simulink model "reglertest2"  (Simulink 7.4)
settings: Solver=ode23  StartTime=0.0  StopTime=1000  MaxStep=0.01  RelTol=1e-3
values from neighbouring files (symbols this model uses):
  KD = polyCOGx    [automatic_controller_2_NOPDT.m]    (also in automatic_controller_2_NOPDT_dycops.m; automatic_controller_NOPDT.m; manual_controller_NOPDT.m = KDa; stable_regions_PID5.m = optimalpolyCOGx)
  KI = polyCOGy    [automatic_controller_2_NOPDT.m]    (also in automatic_controller_2_NOPDT_dycops.m; automatic_controller_NOPDT.m; manual_controller_NOPDT.m = KIa; stable_regions_PID5.m = optimalpolyCOGy)
  KP = KPAmax    [automatic_controller_2_NOPDT.m]    (also in automatic_controller_2_NOPDT_dycops.m; automatic_controller_NOPDT.m = 0.05*KPmax; calc_max_polytope.m = KPvec(i); calc_max_polytope_NO.m = KPvec(i))
  L1 = get(Gref1,'OutputDelay')    [automatic_controller_2_NOPDT.m]    (also in automatic_controller_2_NOPDT_dycops.m)
undefined symbols (not defined in the file or in its folder): Ds1, Ns1
libraries: simulink x3
settings Model: Creator=sle  LastModifiedBy=sle

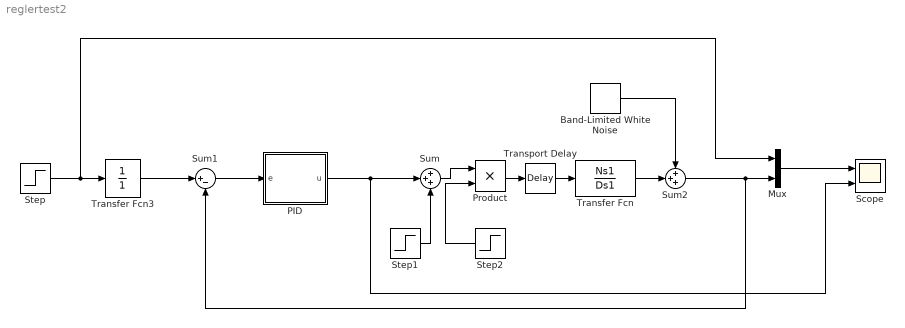
== system reglertest2 ==
  Band-Limited White Noise : simulink/Sources/Band-Limited White Noise  SystemSampleTime=-1  Cov=[0.00001]  Ts=0.1  seed=[23341]
  Mux : Mux  Inputs=2
  PID : Subsystem  mask{KP=KP, KI=KI, KD=KD, Tf=10, OG=900, UG=0}
      mask prompts: Tf "Filterzeitkonstante Tf"; OG "AntiWindup Obergrenze"; UG "AntiWindup Untergrenze"
  Product : Product  OutDataType=fixdt(1, 16)  OutScaling=2^0  RndMeth=Zero
  Scope : Scope  NumInputPorts=2
      settings: YMin=-5~-5  YMax=5~5
  Step : Step  Time=700  Before=1  After=0.5  SampleTime=0
  Step1 : Step  Time=300  After=0.1  SampleTime=0
  Step2 : Step  Time=500  Before=1  After=2  SampleTime=0
  Sum : Sum  Inputs=+++  OutDataType=fixdt(1, 16)  OutScaling=2^0
  Sum1 : Sum  Inputs=|+-  OutDataType=fixdt(1, 16)  OutScaling=2^0
  Sum2 : Sum  Inputs=+++  OutDataType=fixdt(1, 16)  OutScaling=2^0
  Transfer Fcn : TransferFcn  Numerator=Ns1  Denominator=Ds1
  Transfer Fcn3 : TransferFcn  Numerator=1  Denominator=1
  Transport Delay : TransportDelay  DelayTime=L1
  wires:
  Transport Delay/1 -> Transfer Fcn/1
  PID/1(u) -> Sum/2, Scope/2
  Step/1 -> Transfer Fcn3/1, Mux/1
  Mux/1 -> Scope/1
  Step1/1 -> Sum/3
  Sum1/1 -> PID/1(e)
  Transfer Fcn/1 -> Sum2/2
  Sum2/1 -> Mux/2, Sum1/2
  Band-Limited White Noise/1 -> Sum2/1
  Transfer Fcn3/1 -> Sum1/1
  Product/1 -> Transport Delay/1
  Sum/1 -> Product/1
  Step2/1 -> Product/2

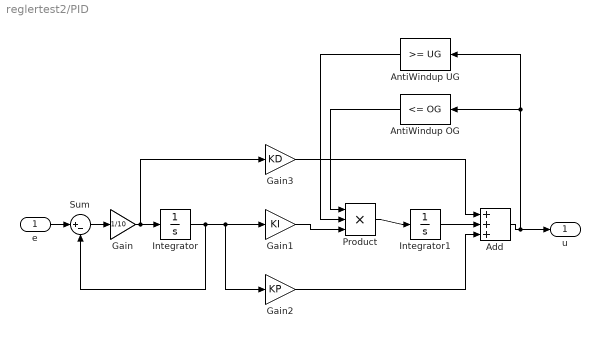
== system reglertest2/PID ==
  e : Inport  OutDataType=fixdt(1, 16)  OutScaling=2^0
  Add : Sum  Inputs=+++  OutDataType=fixdt(1, 16)  OutScaling=2^-10
  AntiWindup OG : simulink/Logic and Bit Operations/Compare To Constant  SystemSampleTime=-1  relop=<=  const=OG  LogicOutDataTypeMode=uint8  ZeroCross=off
  AntiWindup UG : simulink/Logic and Bit Operations/Compare To Constant  SystemSampleTime=-1  relop=>=  const=UG  LogicOutDataTypeMode=uint8  ZeroCross=off
  Gain : Gain  Gain=1/10  ParameterDataType=fixdt(1, 16)  ParameterScaling=2^0  OutDataType=fixdt(1, 16)  OutScaling=2^0
  Gain1 : Gain  Gain=KI  ParameterDataType=fixdt(1, 16)  ParameterScaling=2^0  OutDataType=fixdt(1, 16)  OutScaling=2^0
  Gain2 : Gain  Gain=KP  ParameterDataType=fixdt(1, 16)  ParameterScaling=2^0  OutDataType=fixdt(1, 16)  OutScaling=2^0
  Gain3 : Gain  Gain=KD  ParameterDataType=fixdt(1, 16)  ParameterScaling=2^0  OutDataType=fixdt(1, 16)  OutScaling=2^0
  Integrator : Integrator
  Integrator1 : Integrator
  Product : Product  Inputs=3  OutDataTypeMode=double  OutDataType=fixdt(1, 16)  OutScaling=2^0  OutDataTypeStr=double  RndMeth=Zero
  Sum : Sum  Inputs=|+-  OutDataType=fixdt(1, 16)  OutScaling=2^0
  u : Outport  OutDataType=fixdt(1, 16)  OutScaling=2^0
  wires:
  Add/1 -> u/1, AntiWindup UG/1, AntiWindup OG/1
  e/1 -> Sum/1
  Sum/1 -> Gain/1
  Integrator/1 -> Gain1/1, Gain2/1, Sum/2
  Product/1 -> Integrator1/1
  Integrator1/1 -> Add/2
  Gain2/1 -> Add/3
  Gain3/1 -> Add/1
  Gain1/1 -> Product/3
  AntiWindup UG/1 -> Product/2
  AntiWindup OG/1 -> Product/1
  Gain/1 -> Integrator/1, Gain3/1
